simulink model "tut04"  (R2024a)
settings: Solver=VariableStepAuto  StartTime=0.0  StopTime=10.0  RelTol=1e-3
settings Model: Creator=User  LastModifiedBy=User

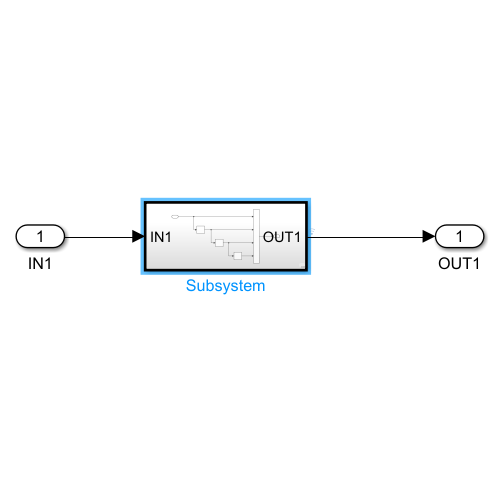
[thumbnail: Simulink's stored preview of the top-level diagram]
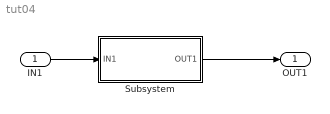
== system tut04 ==
  IN1 : Inport
  Subsystem : Subsystem  TreatAsAtomicUnit=on
  OUT1 : Outport
  wires:
  Subsystem/1(OUT1) -> OUT1/1
  IN1/1 -> Subsystem/1(IN1)

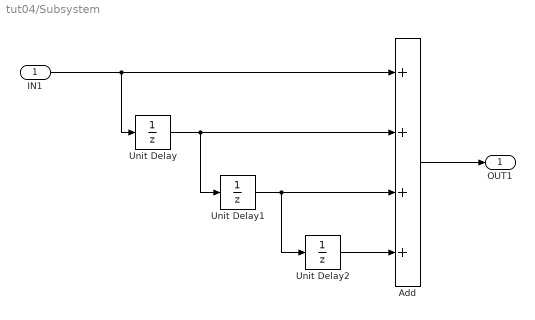
== system tut04/Subsystem ==
  IN1 : Inport
  Add : Sum  Inputs=++++
  Unit Delay : UnitDelay  SampleTime=-1  HasFrameUpgradeWarning=on
  Unit Delay1 : UnitDelay  SampleTime=-1  HasFrameUpgradeWarning=on
  Unit Delay2 : UnitDelay  SampleTime=-1  HasFrameUpgradeWarning=on
  OUT1 : Outport
  wires:
  IN1/1 -> Unit Delay/1, Add/1
  Unit Delay/1 -> Unit Delay1/1, Add/2
  Unit Delay1/1 -> Unit Delay2/1, Add/3
  Unit Delay2/1 -> Add/4
  Add/1 -> OUT1/1
